simulink model "heev_embedded_controller"  (R2015a)
settings: Solver=FixedStepDiscrete  StartTime=0.0  StopTime=10.0  FixedStep=0.005  RelTol=1e-3
PreLoadFcn:
  | try, model_open; catch, disp('Error occurred while executing model pre-load callback: model_open.m'); disp('Please assure that the MATLAB working directory is set to the model directory before opening.'); end
undefined symbols (not defined in the file or in its folder): HCM, raptor_get_safe_string, raptor_xcp_function
libraries: Raptor_lib x37, simulink x2
CloseFcn:
  | try, model_close(bdroot); catch, end
settings Model: Raptor_Target=HCM-5534-90-1302  Raptor_Calloc=NonVolatile (EEPROM)  RaptorUIDSize=4  RaptorBuildNum=1  Creator=Ben  LastModifiedBy=rlamsen
settings DataIOCC: SignalLoggingSaveFormat=ModelDataLogs
settings OptimizationCC: InlineParams=on  ExpressionDepthLimit=2147483647  InitFltsAndDblsToZero=on  OptimizeModelRefInitCode=on  LifeSpan=1
settings DebuggingCC: UnderspecifiedInitializationDetection=Classic  MergeDetectMultiDrivingBlocksExec=none  SolverPrmCheckMsg=warning  InheritedTsInSrcMsg=none  FcnCallInpInsideContextMsg=EnableAllAsWarning  StateNameClashWarn=warning
settings HardwareCC: ProdLargestAtomicInteger=Long  ProdLargestAtomicFloat=Double  ProdIntDivRoundTo=Zero  ProdEndianess=BigEndian  ProdHWDeviceType=Freescale->MPC55xx  TargetLongLongMode=on  TargetIntDivRoundTo=Zero  TargetEndianess=LittleEndian  TargetHWDeviceType=MATLAB Host  ProdEqTarget=off
settings RTWCC: SystemTargetFile=raptor.tlc  MakeCommand=raptor_make_rtw  TemplateMakefile=raptor.tmf  Description=Raptor (tm)
settings CodeAppCC: IgnoreCustomStorageClasses=off  MaxIdLength=100  CustomSymbolStrType=$N$R$M  InternalIdentifier=Classic
settings STFCustomTargetCC: ModelReferenceCompliant=off  CombineOutputUpdateFcns=on  SupportContinuousTime=off  SupportVariableSizeSignals=off  SystemTargetFile=raptor.tlc
settings ERTTargetCC: ModelReferenceCompliant=off  SupportContinuousTime=off  SupportVariableSizeSignals=off  ExtModeMexFile=noextcomm  ERTCustomFileTemplate=example_file_process.tlc

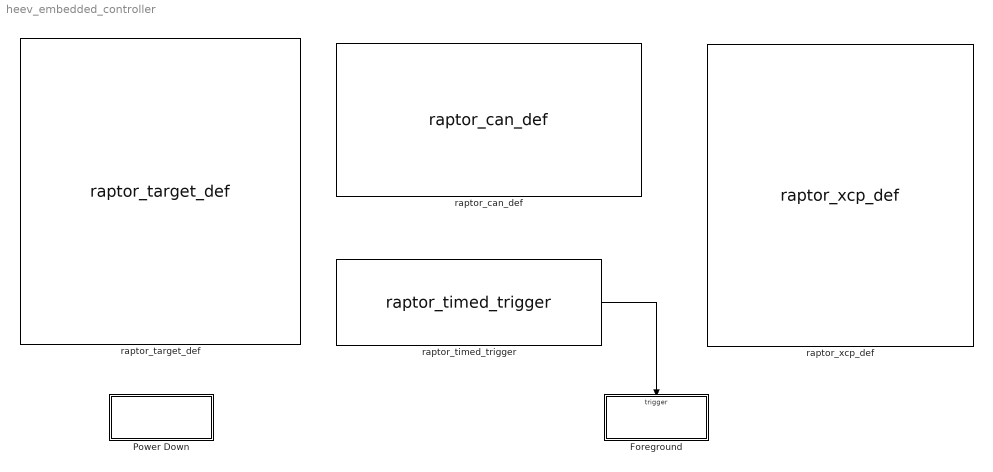
== system heev_embedded_controller ==
  Foreground : Subsystem  TreatAsAtomicUnit=on
  Power Down : Subsystem  TreatAsAtomicUnit=on
  raptor_can_def : Raptor_lib/CAN/raptor_can_def  baudRateValues=250k  baudRate=250k  canBus='CAN1'  resourceValues=(None)|CAN1|CAN2  resource=CAN1
  raptor_target_def : Raptor_lib/Configuration/raptor_target_def  a2lLocation=''  addBuildNum=1  buildLocationValues=Raptor Default|Model Directory|User Defined  buildLocation=Raptor Default  callocValues=Constant (FLASH)|NonVolatile (EEPROM)  calloc=NonVolatile (EEPROM)  compilerValues=CodeWarrior for MPC55xx/MPC56xx Microcontrollers V2.10  compiler=CodeWarrior for MPC55xx/MPC56xx Microcontrollers V2.10  ecuaddr=253  exeLocation=''  exeName=[raptor_get_safe_string(bdroot) '_']  heap=2*1024  minVerChars=3  rpgLocation=''  setFileName=0  simpack=0  simulator=0  stack=2*1024  targetValues=BCM-5646-48-1404|DISP-IMX286-012-1402|DISP-IMX286-024-1204|DISP-IMX286-036-1402|HCM-5534-50-1203|HCM-5534-90-1201|HCM-5534-90-1302|HCM-5604-36-1303|HCM-ARM4-070-1401  target=HCM-5534-90-1302
  raptor_timed_trigger : Raptor_lib/Triggers/raptor_timed_trigger  alwaysEnabled=1  triggerValues=[]  trigger=Foreground  triggerName=ooqlV  triggerPriority=0
  raptor_xcp_def : Raptor_lib/Configuration/raptor_xcp_def  bcID=hex2dec('100')  bcID_TypeValues=[]  bcID_Type=Standard  canBus='CAN1'  daqRates=[5 10 100]  dllName=raptor_XCPSecurity.dll  genCANAPE=0  numODTs=8  rxID=hex2dec('200')  rxID_TypeValues=[]  rxID_Type=Standard  securityValues=[]  security=Standard  txID=hex2dec('300')  txID_TypeValues=[]  txID_Type=Standard
  wires:
  raptor_timed_trigger/1 -> Foreground/Trigger

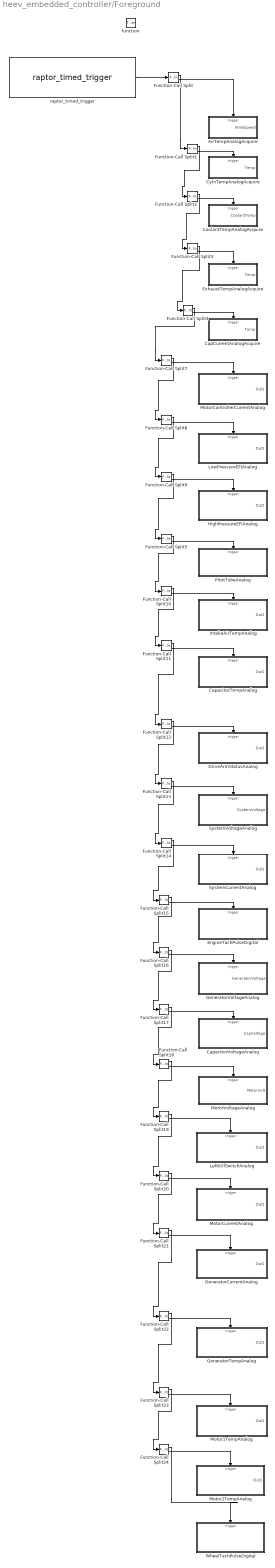
== system heev_embedded_controller/Foreground ==
  function : TriggerPort  TriggerType=function-call
  AirTempAnalogAcquire : Subsystem  TreatAsAtomicUnit=on
  CapCurrentAnalogAcquire : Subsystem  TreatAsAtomicUnit=on
  CapacitorTempAnalog : Subsystem
  CapacitorVoltageAnalog : Subsystem
  CoolantTempAnalogAcquire : Subsystem  TreatAsAtomicUnit=on
  CylnTempAnalogAcquire : Subsystem  TreatAsAtomicUnit=on
  DriveArmStatusAnalog : Subsystem
  EngineTachPulseDigital : Subsystem
  ExhaustTempAnalogAcquire : Subsystem  TreatAsAtomicUnit=on
  Function-Call Split{,1..5,7..24} (24 alike) : FunctionCallSplit
  GeneratorCurrentAnalog : Subsystem
  GeneratorTempAnalog : Subsystem
  GeneratorVoltageAnalog : Subsystem
  HighPressureEFIAnalog : Subsystem
  IntakeAirTempAnalog : Subsystem
  LeftKillSwitchAnalog : Subsystem
  LowPressureEFIAnalog : Subsystem
  Motor1TempAnalog : Subsystem
  Motor2TempAnalog : Subsystem
  MotorControllerCurrentAnalog : Subsystem
  MotorCurrentAnalog : Subsystem
  MotorVoltageAnalog : Subsystem
  PitotTubeAnalog : Subsystem
  SystemCurrentAnalog : Subsystem
  SystemVoltageAnalog : Subsystem
  WheelTachPulseDigital : Subsystem
  raptor_timed_trigger : Raptor_lib/Triggers/raptor_timed_trigger  alwaysEnabled=1  triggerValues=Foreground|Foregroundx2|Foregroundx5|Foregroundx10|Foregroundx20|Background|Backgroundx2|Backgroundx5|Backgroundx10|Backgroundx20|Second|Minute  trigger=Foreground  triggerName=FGND_eMLQ3  triggerPriority=0
  wires:
  Function-Call Split/2 -> AirTempAnalogAcquire/Trigger
  raptor_timed_trigger/1 -> Function-Call Split/1
  Function-Call Split/1 -> Function-Call Split1/1
  Function-Call Split1/2 -> CylnTempAnalogAcquire/Trigger
  Function-Call Split2/2 -> CoolantTempAnalogAcquire/Trigger
  Function-Call Split1/1 -> Function-Call Split2/1
  Function-Call Split3/2 -> ExhaustTempAnalogAcquire/Trigger
  Function-Call Split2/1 -> Function-Call Split3/1
  Function-Call Split4/1 -> Function-Call Split7/1
  Function-Call Split7/2 -> MotorControllerCurrentAnalog/Trigger
  Function-Call Split8/2 -> LowPressureEFIAnalog/Trigger
  Function-Call Split7/1 -> Function-Call Split8/1
  Function-Call Split8/1 -> Function-Call Split9/1
  Function-Call Split9/2 -> HighPressureEFIAnalog/Trigger
  Function-Call Split10/2 -> IntakeAirTempAnalog/Trigger
  Function-Call Split11/2 -> CapacitorTempAnalog/Trigger
  Function-Call Split10/1 -> Function-Call Split11/1
  Function-Call Split12/2 -> DriveArmStatusAnalog/Trigger
  Function-Call Split11/1 -> Function-Call Split12/1
  Function-Call Split13/2 -> SystemVoltageAnalog/Trigger
  Function-Call Split12/1 -> Function-Call Split13/1
  Function-Call Split14/2 -> SystemCurrentAnalog/Trigger
  Function-Call Split13/1 -> Function-Call Split14/1
  Function-Call Split14/1 -> Function-Call Split15/1
  Function-Call Split15/2 -> EngineTachPulseDigital/Trigger
  Function-Call Split15/1 -> Function-Call Split16/1
  Function-Call Split16/2 -> GeneratorVoltageAnalog/Trigger
  Function-Call Split17/2 -> CapacitorVoltageAnalog/Trigger
  Function-Call Split16/1 -> Function-Call Split17/1
  Function-Call Split18/2 -> MotorVoltageAnalog/Trigger
  Function-Call Split17/1 -> Function-Call Split18/1
  Function-Call Split19/2 -> LeftKillSwitchAnalog/Trigger
  Function-Call Split18/1 -> Function-Call Split19/1
  Function-Call Split21/2 -> GeneratorCurrentAnalog/Trigger
  Function-Call Split20/1 -> Function-Call Split21/1
  Function-Call Split19/1 -> Function-Call Split20/1
  Function-Call Split20/2 -> MotorCurrentAnalog/Trigger
  Function-Call Split22/2 -> GeneratorTempAnalog/Trigger
  Function-Call Split21/1 -> Function-Call Split22/1
  Function-Call Split24/2 -> Motor2TempAnalog/Trigger
  Function-Call Split23/1 -> Function-Call Split24/1
  Function-Call Split22/1 -> Function-Call Split23/1
  Function-Call Split23/2 -> Motor1TempAnalog/Trigger
  Function-Call Split24/1 -> WheelTachPulseDigital/Trigger
  Function-Call Split4/2 -> CapCurrentAnalogAcquire/Trigger
  Function-Call Split3/1 -> Function-Call Split4/1
  Function-Call Split5/2 -> PitotTubeAnalog/Trigger
  Function-Call Split9/1 -> Function-Call Split5/1
  Function-Call Split5/1 -> Function-Call Split10/1

== system heev_embedded_controller/Power Down ==
  Subsystem : Subsystem
  raptor_timed_trigger1 : Raptor_lib/Triggers/raptor_timed_trigger  alwaysEnabled=1  triggerValues=Foreground|Foregroundx2|Foregroundx5|Foregroundx10|Foregroundx20|Background|Backgroundx2|Backgroundx5|Backgroundx10|Backgroundx20|Second|Minute  trigger=Background  triggerName=PowerDown  triggerPriority=0
  wires:
  raptor_timed_trigger1/1 -> Subsystem/Trigger

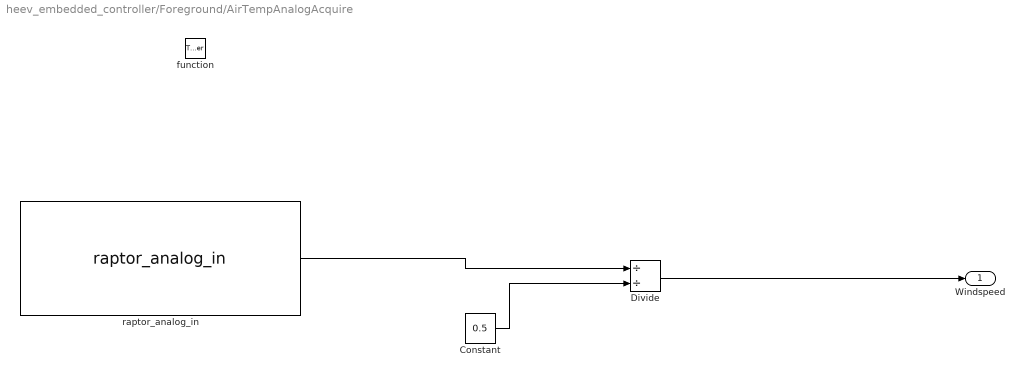
== system heev_embedded_controller/Foreground/AirTempAnalogAcquire ==
  function : TriggerPort  TriggerType=function-call
  Constant : Constant  Value=0.5
  Divide : Product  Inputs=//
  raptor_analog_in : Raptor_lib/Input & Output/raptor_analog_in  filterrateValues=[]  filterrate='RAPTOR MASK DEFAULT'  pullUDValues=None|3.33k PU|3.33k PD|3.33k PU, 3.33k PD  pullUD=None  rangeValues=0 - 38.31 V  range=0 - 38.31 V  resourceValues=(None)|INPUT1|INPUT2|INPUT3|INPUT4|INPUT5|INPUT6|INPUT7|INPUT8|INPUT9|INPUT10|INPUT11|INPUT12|INPUT13|INPUT14|INPUT15|INPUT16|INPUT17|INPUT18|INPUT19|INPUT20|INPUT21|INPUT22|INPUT23|INPUT24|INPUT25|INPUT26|INPUT27|INPUT28|INPUT29|INPUT30|INPUT31|INPUT32|INPUT33|INPUT34|INPUT35|INPUT36  resource=INPUT1
  Windspeed : Outport
  wires:
  raptor_analog_in/1 -> Divide/1
  Divide/1 -> Windspeed/1
  Constant/1 -> Divide/2

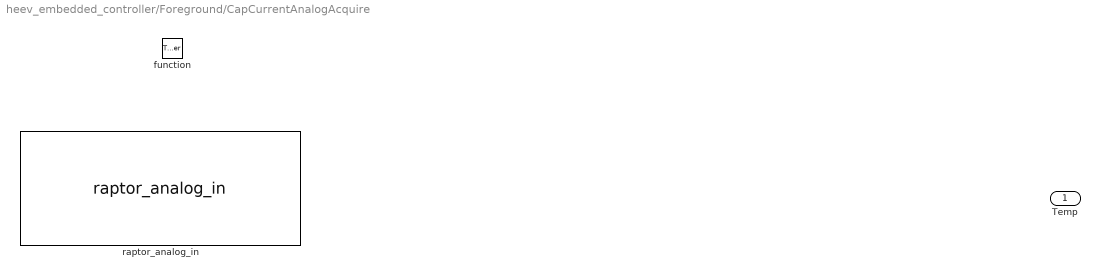
== system heev_embedded_controller/Foreground/CapCurrentAnalogAcquire ==
  function : TriggerPort  TriggerType=function-call  PortDimensions=1
  raptor_analog_in : Raptor_lib/Input & Output/raptor_analog_in  filterrateValues=[]  filterrate='RAPTOR MASK DEFAULT'  pullUDValues=None|650 PU|16.6k PU|50k PD|249 PD  pullUD=None  rangeValues=0 - 4.40 V|0 - 6.49 V|0 - 10.69 V|0 - 12.78 V  range=0 - 4.40 V  resourceValues=(None)|INPUT1|INPUT2|INPUT3|INPUT4|INPUT5|INPUT6|INPUT7|INPUT8|INPUT9|INPUT10|INPUT11|INPUT12|INPUT13|INPUT14|INPUT15|INPUT16|INPUT17|INPUT18|INPUT19|INPUT20|INPUT21|INPUT22|INPUT23|INPUT24|INPUT25|INPUT26|INPUT27|INPUT28|INPUT29|INPUT30|INPUT31|INPUT32|INPUT33|INPUT34|INPUT35|INPUT36  resource=INPUT9
  Temp : Outport

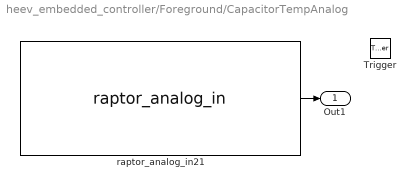
== system heev_embedded_controller/Foreground/CapacitorTempAnalog ==
  Trigger : TriggerPort  TriggerType=function-call  PortDimensions=1
  raptor_analog_in21 : Raptor_lib/Input & Output/raptor_analog_in  filterrateValues=[]  filterrate='RAPTOR MASK DEFAULT'  pullUDValues=None|249 PD  pullUD=None  rangeValues=0 - 22.90 V  range=0 - 22.90 V  resourceValues=(None)|INPUT1|INPUT2|INPUT3|INPUT4|INPUT5|INPUT6|INPUT7|INPUT8|INPUT9|INPUT10|INPUT11|INPUT12|INPUT13|INPUT14|INPUT15|INPUT16|INPUT17|INPUT18|INPUT19|INPUT20|INPUT21|INPUT22|INPUT23|INPUT24|INPUT25|INPUT26|INPUT27|INPUT28|INPUT29|INPUT30|INPUT31|INPUT32|INPUT33|INPUT34|INPUT35|INPUT36  resource=INPUT17
  Out1 : Outport
  wires:
  raptor_analog_in21/1 -> Out1/1

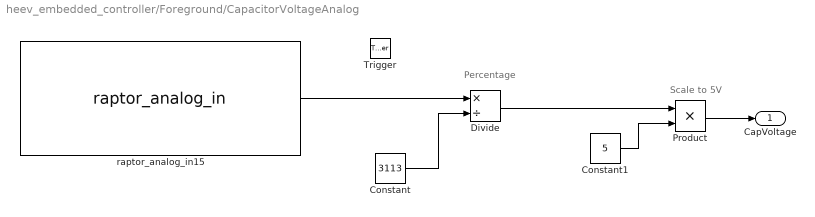
== system heev_embedded_controller/Foreground/CapacitorVoltageAnalog ==
  note: Scale to 5V
  note: Percentage
  Trigger : TriggerPort  TriggerType=function-call  PortDimensions=1
  Constant : Constant  Value=3113  OutDataTypeStr=Inherit: Inherit via back propagation
  Constant1 : Constant  Value=5  OutDataTypeStr=Inherit: Inherit via back propagation
  Divide : Product  Inputs=*/  OutDataTypeStr=double
  Product : Product  OutDataTypeStr=Inherit: Inherit via back propagation
  raptor_analog_in15 : Raptor_lib/Input & Output/raptor_analog_in  filterrateValues=[]  filterrate='RAPTOR MASK DEFAULT'  pullUDValues=None|3.33k PU|3.33k PD|3.33k PU, 3.33k PD  pullUD=None  rangeValues=0 - 38.31 V  range=0 - 38.31 V  resourceValues=(None)|INPUT1|INPUT2|INPUT3|INPUT4|INPUT5|INPUT6|INPUT7|INPUT8|INPUT9|INPUT10|INPUT11|INPUT12|INPUT13|INPUT14|INPUT15|INPUT16|INPUT17|INPUT18|INPUT19|INPUT20|INPUT21|INPUT22|INPUT23|INPUT24|INPUT25|INPUT26|INPUT27|INPUT28|INPUT29|INPUT30|INPUT31|INPUT32|INPUT33|INPUT34|INPUT35|INPUT36  resource=INPUT6
  CapVoltage : Outport
  wires:
  raptor_analog_in15/1 -> Divide/1
  Constant/1 -> Divide/2
  Divide/1 -> Product/1
  Constant1/1 -> Product/2
  Product/1 -> CapVoltage/1

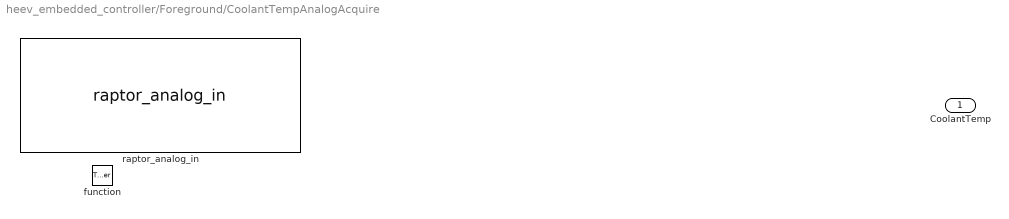
== system heev_embedded_controller/Foreground/CoolantTempAnalogAcquire ==
  function : TriggerPort  TriggerType=function-call  PortDimensions=1
  raptor_analog_in : Raptor_lib/Input & Output/raptor_analog_in  filterrateValues=[]  filterrate='RAPTOR MASK DEFAULT'  pullUDValues=None|3.33k PU|3.33k PD|3.33k PU, 3.33k PD  pullUD=None  rangeValues=0 - 38.31 V  range=0 - 38.31 V  resourceValues=(None)|INPUT1|INPUT2|INPUT3|INPUT4|INPUT5|INPUT6|INPUT7|INPUT8|INPUT9|INPUT10|INPUT11|INPUT12|INPUT13|INPUT14|INPUT15|INPUT16|INPUT17|INPUT18|INPUT19|INPUT20|INPUT21|INPUT22|INPUT23|INPUT24|INPUT25|INPUT26|INPUT27|INPUT28|INPUT29|INPUT30|INPUT31|INPUT32|INPUT33|INPUT34|INPUT35|INPUT36  resource=INPUT3
  CoolantTemp : Outport

== system heev_embedded_controller/Foreground/CylnTempAnalogAcquire ==
  function : TriggerPort  TriggerType=function-call
  raptor_analog_in : Raptor_lib/Input & Output/raptor_analog_in  filterrateValues=[]  filterrate='RAPTOR MASK DEFAULT'  pullUDValues=None|3.33k PU|3.33k PD|3.33k PU, 3.33k PD  pullUD=None  rangeValues=0 - 38.31 V  range=0 - 38.31 V  resourceValues=(None)|INPUT1|INPUT2|INPUT3|INPUT4|INPUT5|INPUT6|INPUT7|INPUT8|INPUT9|INPUT10|INPUT11|INPUT12|INPUT13|INPUT14|INPUT15|INPUT16|INPUT17|INPUT18|INPUT19|INPUT20|INPUT21|INPUT22|INPUT23|INPUT24|INPUT25|INPUT26|INPUT27|INPUT28|INPUT29|INPUT30|INPUT31|INPUT32|INPUT33|INPUT34|INPUT35|INPUT36  resource=INPUT2
  Temp : Outport

== system heev_embedded_controller/Foreground/DriveArmStatusAnalog ==
  Trigger : TriggerPort  TriggerType=function-call  PortDimensions=1
  raptor_analog_in20 : Raptor_lib/Input & Output/raptor_analog_in  filterrateValues=[]  filterrate='RAPTOR MASK DEFAULT'  pullUDValues=None|249 PD  pullUD=None  rangeValues=0 - 22.90 V  range=0 - 22.90 V  resourceValues=(None)|INPUT1|INPUT2|INPUT3|INPUT4|INPUT5|INPUT6|INPUT7|INPUT8|INPUT9|INPUT10|INPUT11|INPUT12|INPUT13|INPUT14|INPUT15|INPUT16|INPUT17|INPUT18|INPUT19|INPUT20|INPUT21|INPUT22|INPUT23|INPUT24|INPUT25|INPUT26|INPUT27|INPUT28|INPUT29|INPUT30|INPUT31|INPUT32|INPUT33|INPUT34|INPUT35|INPUT36  resource=INPUT20
  Out1 : Outport
  wires:
  raptor_analog_in20/1 -> Out1/1

== system heev_embedded_controller/Foreground/EngineTachPulseDigital ==
  Trigger : TriggerPort  TriggerType=function-call  PortDimensions=1
  raptor_can_txraw : Raptor_lib/CAN/raptor_can_txraw  canBus='CAN1'  queueSize=200
  raptor_freq_in : Raptor_lib/Input & Output/raptor_freq_in  filterValues=1kHz|3kHz|10kHz  filter=1kHz  hasDuty=off  hasEdgeCount=off  pullUDValues=4.75k PU, 5.46k PD|5.46k PD  pullUD=4.75k PU, 5.46k PD  resourceValues=(None)|INPUT33|INPUT34|INPUT35|INPUT36  resource=INPUT33

== system heev_embedded_controller/Foreground/ExhaustTempAnalogAcquire ==
  function : TriggerPort  TriggerType=function-call  PortDimensions=1
  raptor_analog_in : Raptor_lib/Input & Output/raptor_analog_in  filterrateValues=[]  filterrate='RAPTOR MASK DEFAULT'  pullUDValues=None|3.33k PU|3.33k PD|3.33k PU, 3.33k PD  pullUD=None  rangeValues=0 - 38.31 V  range=0 - 38.31 V  resourceValues=(None)|INPUT1|INPUT2|INPUT3|INPUT4|INPUT5|INPUT6|INPUT7|INPUT8|INPUT9|INPUT10|INPUT11|INPUT12|INPUT13|INPUT14|INPUT15|INPUT16|INPUT17|INPUT18|INPUT19|INPUT20|INPUT21|INPUT22|INPUT23|INPUT24|INPUT25|INPUT26|INPUT27|INPUT28|INPUT29|INPUT30|INPUT31|INPUT32|INPUT33|INPUT34|INPUT35|INPUT36  resource=INPUT4
  Temp : Outport

== system heev_embedded_controller/Foreground/GeneratorCurrentAnalog ==
  Trigger : TriggerPort  TriggerType=function-call  PortDimensions=1
  raptor_analog_in11 : Raptor_lib/Input & Output/raptor_analog_in  filterrateValues=[]  filterrate='RAPTOR MASK DEFAULT'  pullUDValues=None|650 PU|16.6k PU|50k PD|249 PD  pullUD=None  rangeValues=0 - 4.40 V|0 - 6.49 V|0 - 10.69 V|0 - 12.78 V  range=0 - 4.40 V  resourceValues=(None)|INPUT1|INPUT2|INPUT3|INPUT4|INPUT5|INPUT6|INPUT7|INPUT8|INPUT9|INPUT10|INPUT11|INPUT12|INPUT13|INPUT14|INPUT15|INPUT16|INPUT17|INPUT18|INPUT19|INPUT20|INPUT21|INPUT22|INPUT23|INPUT24|INPUT25|INPUT26|INPUT27|INPUT28|INPUT29|INPUT30|INPUT31|INPUT32|INPUT33|INPUT34|INPUT35|INPUT36  resource=INPUT12
  Out1 : Outport
  wires:
  raptor_analog_in11/1 -> Out1/1

== system heev_embedded_controller/Foreground/GeneratorTempAnalog ==
  Trigger : TriggerPort  TriggerType=function-call  PortDimensions=1
  raptor_analog_in10 : Raptor_lib/Input & Output/raptor_analog_in  filterrateValues=[]  filterrate='RAPTOR MASK DEFAULT'  pullUDValues=None|249 PD  pullUD=None  rangeValues=0 - 22.90 V  range=0 - 22.90 V  resourceValues=(None)|INPUT1|INPUT2|INPUT3|INPUT4|INPUT5|INPUT6|INPUT7|INPUT8|INPUT9|INPUT10|INPUT11|INPUT12|INPUT13|INPUT14|INPUT15|INPUT16|INPUT17|INPUT18|INPUT19|INPUT20|INPUT21|INPUT22|INPUT23|INPUT24|INPUT25|INPUT26|INPUT27|INPUT28|INPUT29|INPUT30|INPUT31|INPUT32|INPUT33|INPUT34|INPUT35|INPUT36  resource=INPUT28
  Out1 : Outport
  wires:
  raptor_analog_in10/1 -> Out1/1

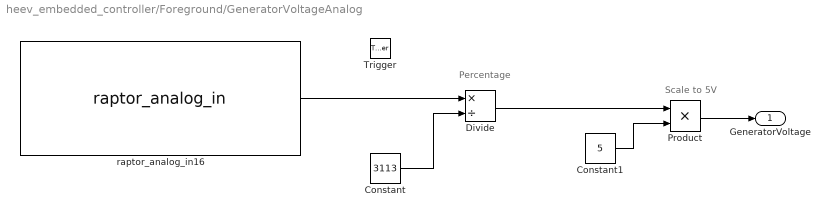
== system heev_embedded_controller/Foreground/GeneratorVoltageAnalog ==
  note: Scale to 5V
  note: Percentage
  Trigger : TriggerPort  TriggerType=function-call  PortDimensions=1
  Constant : Constant  Value=3113  OutDataTypeStr=Inherit: Inherit via back propagation
  Constant1 : Constant  Value=5  OutDataTypeStr=Inherit: Inherit via back propagation
  Divide : Product  Inputs=*/  OutDataTypeStr=double
  Product : Product  OutDataTypeStr=Inherit: Inherit via back propagation
  raptor_analog_in16 : Raptor_lib/Input & Output/raptor_analog_in  filterrateValues=[]  filterrate='RAPTOR MASK DEFAULT'  pullUDValues=None|3.33k PU|3.33k PD|3.33k PU, 3.33k PD  pullUD=None  rangeValues=0 - 38.31 V  range=0 - 38.31 V  resourceValues=(None)|INPUT1|INPUT2|INPUT3|INPUT4|INPUT5|INPUT6|INPUT7|INPUT8|INPUT9|INPUT10|INPUT11|INPUT12|INPUT13|INPUT14|INPUT15|INPUT16|INPUT17|INPUT18|INPUT19|INPUT20|INPUT21|INPUT22|INPUT23|INPUT24|INPUT25|INPUT26|INPUT27|INPUT28|INPUT29|INPUT30|INPUT31|INPUT32|INPUT33|INPUT34|INPUT35|INPUT36  resource=INPUT5
  GeneratorVoltage : Outport
  wires:
  raptor_analog_in16/1 -> Divide/1
  Constant/1 -> Divide/2
  Divide/1 -> Product/1
  Constant1/1 -> Product/2
  Product/1 -> GeneratorVoltage/1

== system heev_embedded_controller/Foreground/HighPressureEFIAnalog ==
  Trigger : TriggerPort  TriggerType=function-call  PortDimensions=1
  raptor_analog_in4 : Raptor_lib/Input & Output/raptor_analog_in  filterrateValues=[]  filterrate='RAPTOR MASK DEFAULT'  pullUDValues=None|249 PD  pullUD=None  rangeValues=0 - 22.90 V  range=0 - 22.90 V  resourceValues=(None)|INPUT1|INPUT2|INPUT3|INPUT4|INPUT5|INPUT6|INPUT7|INPUT8|INPUT9|INPUT10|INPUT11|INPUT12|INPUT13|INPUT14|INPUT15|INPUT16|INPUT17|INPUT18|INPUT19|INPUT20|INPUT21|INPUT22|INPUT23|INPUT24|INPUT25|INPUT26|INPUT27|INPUT28|INPUT29|INPUT30|INPUT31|INPUT32|INPUT33|INPUT34|INPUT35|INPUT36  resource=INPUT14
  Out1 : Outport
  wires:
  raptor_analog_in4/1 -> Out1/1

== system heev_embedded_controller/Foreground/IntakeAirTempAnalog ==
  Trigger : TriggerPort  TriggerType=function-call  PortDimensions=1
  raptor_analog_in3 : Raptor_lib/Input & Output/raptor_analog_in  filterrateValues=[]  filterrate='RAPTOR MASK DEFAULT'  pullUDValues=None|249 PD  pullUD=None  rangeValues=0 - 22.90 V  range=0 - 22.90 V  resourceValues=(None)|INPUT1|INPUT2|INPUT3|INPUT4|INPUT5|INPUT6|INPUT7|INPUT8|INPUT9|INPUT10|INPUT11|INPUT12|INPUT13|INPUT14|INPUT15|INPUT16|INPUT17|INPUT18|INPUT19|INPUT20|INPUT21|INPUT22|INPUT23|INPUT24|INPUT25|INPUT26|INPUT27|INPUT28|INPUT29|INPUT30|INPUT31|INPUT32|INPUT33|INPUT34|INPUT35|INPUT36  resource=INPUT16
  Out1 : Outport
  wires:
  raptor_analog_in3/1 -> Out1/1

== system heev_embedded_controller/Foreground/LeftKillSwitchAnalog ==
  Trigger : TriggerPort  TriggerType=function-call  PortDimensions=1
  raptor_analog_in13 : Raptor_lib/Input & Output/raptor_analog_in  filterrateValues=[]  filterrate='RAPTOR MASK DEFAULT'  pullUDValues=None|3.33k PU|3.33k PD|3.33k PU, 3.33k PD  pullUD=None  rangeValues=0 - 38.31 V  range=0 - 38.31 V  resourceValues=(None)|INPUT1|INPUT2|INPUT3|INPUT4|INPUT5|INPUT6|INPUT7|INPUT8|INPUT9|INPUT10|INPUT11|INPUT12|INPUT13|INPUT14|INPUT15|INPUT16|INPUT17|INPUT18|INPUT19|INPUT20|INPUT21|INPUT22|INPUT23|INPUT24|INPUT25|INPUT26|INPUT27|INPUT28|INPUT29|INPUT30|INPUT31|INPUT32|INPUT33|INPUT34|INPUT35|INPUT36  resource=INPUT8
  Out1 : Outport
  wires:
  raptor_analog_in13/1 -> Out1/1

== system heev_embedded_controller/Foreground/LowPressureEFIAnalog ==
  Trigger : TriggerPort  TriggerType=function-call  PortDimensions=1
  raptor_analog_in5 : Raptor_lib/Input & Output/raptor_analog_in  filterrateValues=[]  filterrate='RAPTOR MASK DEFAULT'  pullUDValues=None|249 PD  pullUD=None  rangeValues=0 - 22.90 V  range=0 - 22.90 V  resourceValues=(None)|INPUT1|INPUT2|INPUT3|INPUT4|INPUT5|INPUT6|INPUT7|INPUT8|INPUT9|INPUT10|INPUT11|INPUT12|INPUT13|INPUT14|INPUT15|INPUT16|INPUT17|INPUT18|INPUT19|INPUT20|INPUT21|INPUT22|INPUT23|INPUT24|INPUT25|INPUT26|INPUT27|INPUT28|INPUT29|INPUT30|INPUT31|INPUT32|INPUT33|INPUT34|INPUT35|INPUT36  resource=INPUT13
  Out1 : Outport
  wires:
  raptor_analog_in5/1 -> Out1/1

== system heev_embedded_controller/Foreground/Motor1TempAnalog ==
  Trigger : TriggerPort  TriggerType=function-call  PortDimensions=1
  raptor_analog_in9 : Raptor_lib/Input & Output/raptor_analog_in  filterrateValues=[]  filterrate='RAPTOR MASK DEFAULT'  pullUDValues=None|249 PD  pullUD=None  rangeValues=0 - 22.90 V  range=0 - 22.90 V  resourceValues=(None)|INPUT1|INPUT2|INPUT3|INPUT4|INPUT5|INPUT6|INPUT7|INPUT8|INPUT9|INPUT10|INPUT11|INPUT12|INPUT13|INPUT14|INPUT15|INPUT16|INPUT17|INPUT18|INPUT19|INPUT20|INPUT21|INPUT22|INPUT23|INPUT24|INPUT25|INPUT26|INPUT27|INPUT28|INPUT29|INPUT30|INPUT31|INPUT32|INPUT33|INPUT34|INPUT35|INPUT36  resource=INPUT31
  Out1 : Outport
  wires:
  raptor_analog_in9/1 -> Out1/1

== system heev_embedded_controller/Foreground/Motor2TempAnalog ==
  Trigger : TriggerPort  TriggerType=function-call  PortDimensions=1
  raptor_analog_in1 : Raptor_lib/Input & Output/raptor_analog_in  filterrateValues=[]  filterrate='RAPTOR MASK DEFAULT'  pullUDValues=None|249 PD  pullUD=None  rangeValues=0 - 22.90 V  range=0 - 22.90 V  resourceValues=(None)|INPUT1|INPUT2|INPUT3|INPUT4|INPUT5|INPUT6|INPUT7|INPUT8|INPUT9|INPUT10|INPUT11|INPUT12|INPUT13|INPUT14|INPUT15|INPUT16|INPUT17|INPUT18|INPUT19|INPUT20|INPUT21|INPUT22|INPUT23|INPUT24|INPUT25|INPUT26|INPUT27|INPUT28|INPUT29|INPUT30|INPUT31|INPUT32|INPUT33|INPUT34|INPUT35|INPUT36  resource=INPUT32
  Out1 : Outport
  wires:
  raptor_analog_in1/1 -> Out1/1

== system heev_embedded_controller/Foreground/MotorControllerCurrentAnalog ==
  Trigger : TriggerPort  TriggerType=function-call  PortDimensions=1
  raptor_analog_in6 : Raptor_lib/Input & Output/raptor_analog_in  filterrateValues=[]  filterrate='RAPTOR MASK DEFAULT'  pullUDValues=None|650 PU|16.6k PU|50k PD|249 PD  pullUD=None  rangeValues=0 - 4.40 V|0 - 6.49 V|0 - 10.69 V|0 - 12.78 V  range=0 - 6.49 V  resourceValues=(None)|INPUT1|INPUT2|INPUT3|INPUT4|INPUT5|INPUT6|INPUT7|INPUT8|INPUT9|INPUT10|INPUT11|INPUT12|INPUT13|INPUT14|INPUT15|INPUT16|INPUT17|INPUT18|INPUT19|INPUT20|INPUT21|INPUT22|INPUT23|INPUT24|INPUT25|INPUT26|INPUT27|INPUT28|INPUT29|INPUT30|INPUT31|INPUT32|INPUT33|INPUT34|INPUT35|INPUT36  resource=INPUT10
  Out1 : Outport
  wires:
  raptor_analog_in6/1 -> Out1/1

== system heev_embedded_controller/Foreground/MotorCurrentAnalog ==
  Trigger : TriggerPort  TriggerType=function-call  PortDimensions=1
  raptor_analog_in12 : Raptor_lib/Input & Output/raptor_analog_in  filterrateValues=[]  filterrate='RAPTOR MASK DEFAULT'  pullUDValues=None|650 PU|16.6k PU|50k PD|249 PD  pullUD=None  rangeValues=0 - 4.40 V|0 - 6.49 V|0 - 10.69 V|0 - 12.78 V  range=0 - 4.40 V  resourceValues=(None)|INPUT1|INPUT2|INPUT3|INPUT4|INPUT5|INPUT6|INPUT7|INPUT8|INPUT9|INPUT10|INPUT11|INPUT12|INPUT13|INPUT14|INPUT15|INPUT16|INPUT17|INPUT18|INPUT19|INPUT20|INPUT21|INPUT22|INPUT23|INPUT24|INPUT25|INPUT26|INPUT27|INPUT28|INPUT29|INPUT30|INPUT31|INPUT32|INPUT33|INPUT34|INPUT35|INPUT36  resource=INPUT11
  Out1 : Outport
  wires:
  raptor_analog_in12/1 -> Out1/1

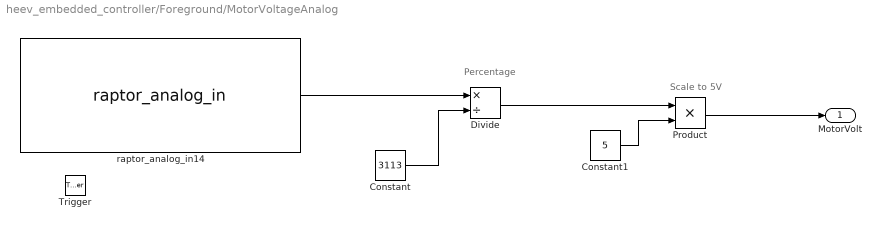
== system heev_embedded_controller/Foreground/MotorVoltageAnalog ==
  note: Scale to 5V
  note: Percentage
  Trigger : TriggerPort  TriggerType=function-call  PortDimensions=1
  Constant : Constant  Value=3113  OutDataTypeStr=Inherit: Inherit via back propagation
  Constant1 : Constant  Value=5  OutDataTypeStr=Inherit: Inherit via back propagation
  Divide : Product  Inputs=*/  OutDataTypeStr=double
  Product : Product  OutDataTypeStr=Inherit: Inherit via back propagation
  raptor_analog_in14 : Raptor_lib/Input & Output/raptor_analog_in  filterrateValues=[]  filterrate='RAPTOR MASK DEFAULT'  pullUDValues=None|3.33k PU|3.33k PD|3.33k PU, 3.33k PD  pullUD=None  rangeValues=0 - 38.31 V  range=0 - 38.31 V  resourceValues=(None)|INPUT1|INPUT2|INPUT3|INPUT4|INPUT5|INPUT6|INPUT7|INPUT8|INPUT9|INPUT10|INPUT11|INPUT12|INPUT13|INPUT14|INPUT15|INPUT16|INPUT17|INPUT18|INPUT19|INPUT20|INPUT21|INPUT22|INPUT23|INPUT24|INPUT25|INPUT26|INPUT27|INPUT28|INPUT29|INPUT30|INPUT31|INPUT32|INPUT33|INPUT34|INPUT35|INPUT36  resource=INPUT7
  MotorVolt : Outport
  wires:
  raptor_analog_in14/1 -> Divide/1
  Constant/1 -> Divide/2
  Divide/1 -> Product/1
  Constant1/1 -> Product/2
  Product/1 -> MotorVolt/1

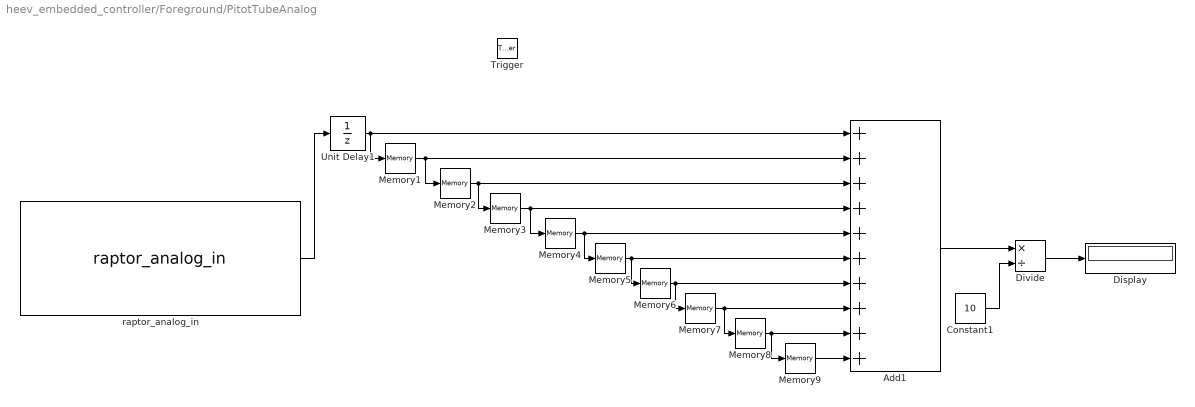
== system heev_embedded_controller/Foreground/PitotTubeAnalog ==
  Trigger : TriggerPort  TriggerType=function-call  PortDimensions=1
  Add1 : Sum  Inputs=++++++++++  OutDataTypeStr=uint16
  Constant1 : Constant  Value=10  VectorParams1D=off  OutDataTypeStr=uint16  LockScale=on
  Display : Display
  Divide : Product  Inputs=*/  OutDataTypeStr=uint16  InputSameDT=on
  Memory{1..9} (9 alike) : Memory  InheritSampleTime=on  LinearizeAsDelay=on
  Unit Delay1 : UnitDelay  SampleTime=-1
  raptor_analog_in : Raptor_lib/Input & Output/raptor_analog_in  filterrateValues=[]  filterrate='RAPTOR MASK DEFAULT'  pullUDValues=None|249 PD  pullUD=None  rangeValues=0 - 22.90 V  range=0 - 22.90 V  resourceValues=(None)|INPUT1|INPUT2|INPUT3|INPUT4|INPUT5|INPUT6|INPUT7|INPUT8|INPUT9|INPUT10|INPUT11|INPUT12|INPUT13|INPUT14|INPUT15|INPUT16|INPUT17|INPUT18|INPUT19|INPUT20|INPUT21|INPUT22|INPUT23|INPUT24|INPUT25|INPUT26|INPUT27|INPUT28|INPUT29|INPUT30|INPUT31|INPUT32|INPUT33|INPUT34|INPUT35|INPUT36  resource=INPUT15
  wires:
  raptor_analog_in/1 -> Unit Delay1/1
  Memory4/1 -> Memory5/1, Add1/5
  Memory2/1 -> Add1/3, Memory3/1
  Memory8/1 -> Add1/9, Memory9/1
  Constant1/1 -> Divide/2
  Add1/1 -> Divide/1
  Memory5/1 -> Memory6/1, Add1/6
  Memory6/1 -> Memory7/1, Add1/7
  Unit Delay1/1 -> Add1/1, Memory1/1
  Memory3/1 -> Add1/4, Memory4/1
  Memory7/1 -> Memory8/1, Add1/8
  Memory1/1 -> Add1/2, Memory2/1
  Memory9/1 -> Add1/10
  Divide/1 -> Display/1

== system heev_embedded_controller/Foreground/SystemCurrentAnalog ==
  Trigger : TriggerPort  TriggerType=function-call  PortDimensions=1
  raptor_analog_in18 : Raptor_lib/Input & Output/raptor_analog_in  filterrateValues=[]  filterrate='RAPTOR MASK DEFAULT'  pullUDValues=None|249 PD  pullUD=None  rangeValues=0 - 22.90 V  range=0 - 22.90 V  resourceValues=(None)|INPUT1|INPUT2|INPUT3|INPUT4|INPUT5|INPUT6|INPUT7|INPUT8|INPUT9|INPUT10|INPUT11|INPUT12|INPUT13|INPUT14|INPUT15|INPUT16|INPUT17|INPUT18|INPUT19|INPUT20|INPUT21|INPUT22|INPUT23|INPUT24|INPUT25|INPUT26|INPUT27|INPUT28|INPUT29|INPUT30|INPUT31|INPUT32|INPUT33|INPUT34|INPUT35|INPUT36  resource=INPUT22
  Out1 : Outport
  wires:
  raptor_analog_in18/1 -> Out1/1

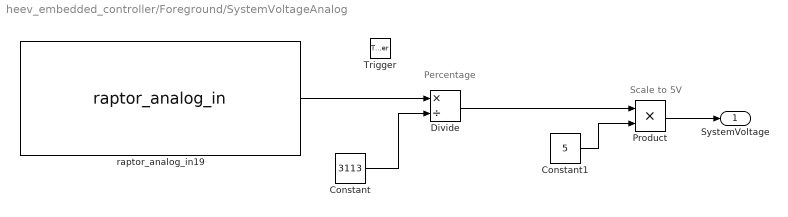
== system heev_embedded_controller/Foreground/SystemVoltageAnalog ==
  note: Scale to 5V
  note: Percentage
  Trigger : TriggerPort  TriggerType=function-call  PortDimensions=1
  Constant : Constant  Value=3113  OutDataTypeStr=Inherit: Inherit via back propagation
  Constant1 : Constant  Value=5  OutDataTypeStr=Inherit: Inherit via back propagation
  Divide : Product  Inputs=*/  OutDataTypeStr=double
  Product : Product  OutDataTypeStr=Inherit: Inherit via back propagation
  raptor_analog_in19 : Raptor_lib/Input & Output/raptor_analog_in  filterrateValues=[]  filterrate='RAPTOR MASK DEFAULT'  pullUDValues=None|249 PD  pullUD=None  rangeValues=0 - 22.90 V  range=0 - 22.90 V  resourceValues=(None)|INPUT1|INPUT2|INPUT3|INPUT4|INPUT5|INPUT6|INPUT7|INPUT8|INPUT9|INPUT10|INPUT11|INPUT12|INPUT13|INPUT14|INPUT15|INPUT16|INPUT17|INPUT18|INPUT19|INPUT20|INPUT21|INPUT22|INPUT23|INPUT24|INPUT25|INPUT26|INPUT27|INPUT28|INPUT29|INPUT30|INPUT31|INPUT32|INPUT33|INPUT34|INPUT35|INPUT36  resource=INPUT21
  SystemVoltage : Outport
  wires:
  raptor_analog_in19/1 -> Divide/1
  Constant/1 -> Divide/2
  Divide/1 -> Product/1
  Constant1/1 -> Product/2
  Product/1 -> SystemVoltage/1

== system heev_embedded_controller/Foreground/WheelTachPulseDigital ==
  Trigger : TriggerPort  TriggerType=function-call  PortDimensions=1
  raptor_freq_in : Raptor_lib/Input & Output/raptor_freq_in  filterValues=1kHz|3kHz|10kHz  filter=1kHz  hasDuty=off  hasEdgeCount=off  pullUDValues=4.75k PU, 5.46k PD|5.46k PD  pullUD=4.75k PU, 5.46k PD  resourceValues=(None)|INPUT33|INPUT34|INPUT35|INPUT36  resource=INPUT35

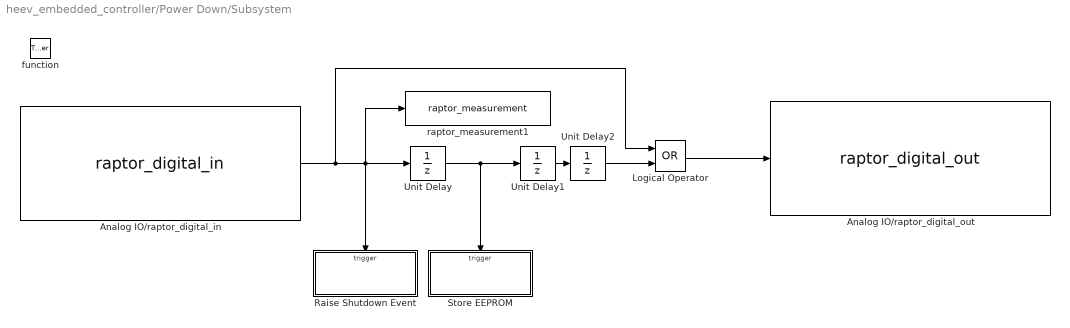
== system heev_embedded_controller/Power Down/Subsystem ==
  function : TriggerPort  TriggerType=function-call
  Analog IO/raptor_digital_in : Raptor_lib/Input & Output/raptor_digital_in  lowerThres=1.320  pullUDValues=2k PD  pullUD=220k PD  resourceValues=(None)|WAKE_INPUT1|INPUT2|INPUT3|INPUT4|INPUT5|INPUT6|INPUT8|INPUT9|INPUT10|INPUT11|INPUT12|INPUT13|INPUT14|INPUT15|INPUT16|INPUT17|INPUT18|INPUT19|INPUT20|INPUT21  resource=WAKE_INPUT1  upperThres=1.980
  Analog IO/raptor_digital_out : Raptor_lib/Input & Output/raptor_digital_out  driverTypeValues=(None)  driverType=(None)  resourceValues=(None)|OUTPUT1|OUTPUT2|OUTPUT3|OUTPUT4|OUTPUT5|OUTPUT6|OUTPUT7|OUTPUT8|OUTPUT9|OUTPUT10|OUTPUT11|OUTPUT12|OUTPUT13|OUTPUT14|OUTPUT15|LED_1|LED_2|LED_3|LED_4|LED_5|LED_6|LED_7|LED_8|LED_9|LED_10|LED_11|LED_12|LED_13|LED_14|LED_15|LED_16|LED_17|LED_18|LED_19|LED_20|LED_21|LED_22|LED_23|LED_24|LED_25|LED_26|LED_27|LED_28|LED_29|LED_30|LED_31|LED_32|LED_33|LED_34|LED_35|LED_36|LED_37|LED_38|LED_39|LED_40|POWER_HOLD|SENS_PWR_EN|SENS_PWR_SEL  resource=POWER_HOLD
  Logical Operator : Logic  Operator=OR  AllPortsSameDT=off  OutDataTypeStr=boolean
  Raise Shutdown Event : Subsystem  TreatAsAtomicUnit=on
  Store EEPROM : Subsystem  TreatAsAtomicUnit=on
  Unit Delay : UnitDelay  SampleTime=-1
  Unit Delay1 : UnitDelay  SampleTime=-1
  Unit Delay2 : UnitDelay  SampleTime=-1
  raptor_measurement1 : Raptor_lib/Data Storage/raptor_measurement  paramName='WakeInput'  nameSource=Parameter  calDispType=Number  calEnum={'False', 'True'}  calGain=1.0  calOffset=0.0  calMax=inf  calMin=-inf  calFormat='-1'  calUnit=''  calHelp=''  calAccess=4  calFunction=raptor_xcp_function(gcb)  calVisible=on
  wires:
  Unit Delay1/1 -> Unit Delay2/1
  Unit Delay/1 -> Unit Delay1/1, Store EEPROM/Trigger
  Analog IO/raptor_digital_in/1 -> Unit Delay/1, Raise Shutdown Event/Trigger, raptor_measurement1/1, Logical Operator/1
  Unit Delay2/1 -> Logical Operator/2
  Logical Operator/1 -> Analog IO/raptor_digital_out/1

== system heev_embedded_controller/Power Down/Subsystem/Raise Shutdown Event ==
  function : TriggerPort  TriggerType=falling
  Function-Call Generator : simulink/Ports & Subsystems/Function-Call Generator  sample_time=-1  numberOfIterations=1
  raptor_shutdown : Raptor_lib/Triggers/raptor_shutdown  null=0
  wires:
  Function-Call Generator/1 -> raptor_shutdown/Trigger

== system heev_embedded_controller/Power Down/Subsystem/Store EEPROM ==
  function : TriggerPort  TriggerType=falling
  Function-Call Generator : simulink/Ports & Subsystems/Function-Call Generator  sample_time=-1  numberOfIterations=1
  raptor_store_nv : Raptor_lib/Data Storage/raptor_store_nv  null=0
  wires:
  Function-Call Generator/1 -> raptor_store_nv/Trigger
